simulink model "Simulink_Encoder"  (R2023b)
settings: Solver=FixedStepAuto  StartTime=0.0  StopTime=10  RelTol=1e-3
undefined symbols (not defined in the file): DiscIntNeverNeededParam
libraries: simulink x3
settings Model: Creator=rodri  LastModifiedBy=rodri

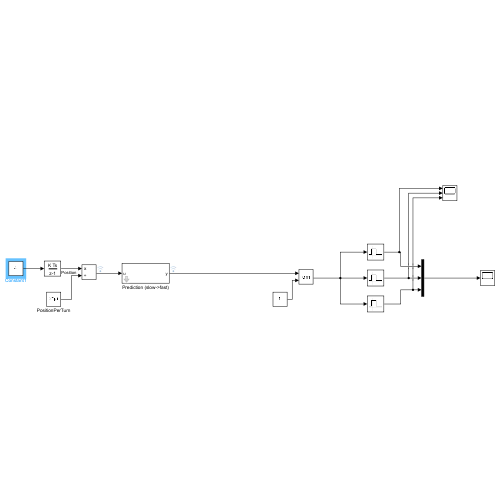
[thumbnail: Simulink's stored preview of the top-level diagram]
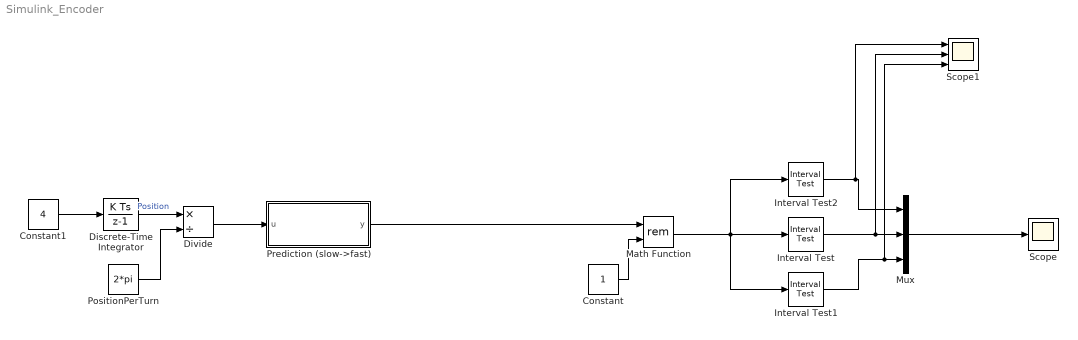
== system Simulink_Encoder ==
  Constant : Constant
  Constant1 : Constant  Value=4  SampleTime=0.1
  Discrete-Time Integrator : DiscreteIntegrator  SampleTime=-1  ICPrevOutput=DiscIntNeverNeededParam  ICPrevScaledInput=DiscIntNeverNeededParam
  Divide : Product  Inputs=*/  RndMeth=Simplest
  Interval Test : simulink/Logic and Bit Operations/Interval Test  IntervalClosedRight=on  uplimit=1  IntervalClosedLeft=on  lowlimit=0.5  OutDataTypeStr=boolean
  Interval Test1 : simulink/Logic and Bit Operations/Interval Test  IntervalClosedRight=on  uplimit=0.125  IntervalClosedLeft=on  lowlimit=0  OutDataTypeStr=boolean
  Interval Test2 : simulink/Logic and Bit Operations/Interval Test  IntervalClosedRight=on  uplimit=0.5  IntervalClosedLeft=on  lowlimit=0  OutDataTypeStr=boolean
  Math Function : Math  Operator=rem
  Mux : Mux  Inputs=3
  PositionPerTurn : Constant  Value=2*pi
  Prediction (slow->fast) : Subsystem  mask(Prediction (slow->fast)){h2=0.1, h1=0.001}
      mask prompts: h2 "physmod:simscape:couplers:SimscapeNetworkCouplersLib:PortUDiscreteSampleTimes_MP"; h1 "physmod:simscape:couplers:SimscapeNetworkCouplersLib:PortYDiscreteSampleTimes_MP"
      mask help: physmod:simscape:couplers:SimscapeNetworkCouplersLib:Predictionslowfast_MD
      mask Help: web([docroot '/simscape/ref/predictionslowfast.html'])
      mask DialogControl h2 Prompt: Port u discrete sample time (s)
      mask DialogControl h1 Prompt: Port y discrete sample time (s)
  Scope : Scope
  Scope1 : Scope  NumInputPorts=3
  wires:
  Mux/1 -> Scope/1
  PositionPerTurn/1 -> Divide/2
  Discrete-Time Integrator/1 -> Divide/1  "Position"
  Constant/1 -> Math Function/2
  Prediction (slow->fast)/1(y) -> Math Function/1
  Math Function/1 -> Interval Test1/1, Interval Test/1, Interval Test2/1
  Interval Test2/1 -> Scope1/1, Mux/1
  Interval Test/1 -> Scope1/2, Mux/2
  Interval Test1/1 -> Scope1/3, Mux/3
  Divide/1 -> Prediction (slow->fast)/1(u)
  Constant1/1 -> Discrete-Time Integrator/1

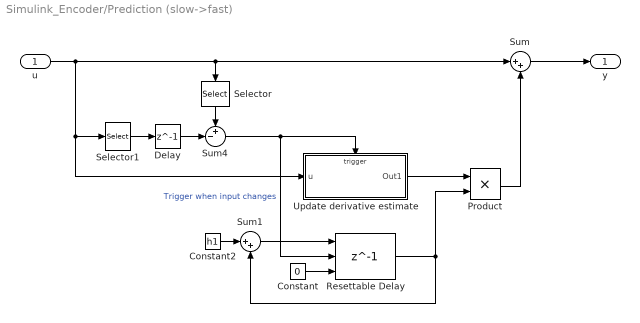
== system Simulink_Encoder/Prediction (slow->fast) ==
  u : Inport
  Constant : Constant  Value=0  SampleTime=h1
  Constant2 : Constant  Value=h1  SampleTime=h1
  "Delay " : Delay  DelayLength=1  SampleTime=h1
  Product : Product
  Resettable Delay : Delay  DelayLength=1  InitialConditionSource=Input port  ExternalReset=Rising  SampleTime=h1
      settings: InputPortMap=u0,r5,p4
  Selector : Selector  IndexOptions=Index vector (dialog)  Indices=1  OutputSizes=1
  Selector1 : Selector  IndexOptions=Index vector (dialog)  Indices=1  OutputSizes=1
  Sum : Sum  Inputs=|++
  Sum1 : Sum  Inputs=|++
  Sum4 : Sum  Inputs=+-|
  Update derivative estimate : Subsystem  TreatAsAtomicUnit=on
  y : Outport
  wires:
  Selector1/1 -> "Delay "/1
  Selector/1 -> Sum4/1
  Product/1 -> Sum/2
  Sum/1 -> y/1
  Constant/1 -> Resettable Delay/3
  Constant2/1 -> Sum1/1
  Resettable Delay/1 -> Sum1/2, Product/2
  Sum1/1 -> Resettable Delay/1
  Sum4/1 -> Resettable Delay/2, Update derivative estimate/Trigger  "Trigger when input changes"
  "Delay "/1 -> Sum4/2
  u/1 -> Sum/1, Selector/1, Update derivative estimate/1(u), Selector1/1
  Update derivative estimate/1(Out1) -> Product/1

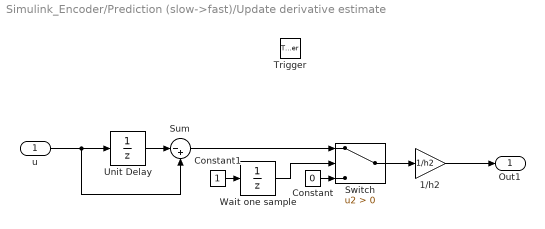
== system Simulink_Encoder/Prediction (slow->fast)/Update derivative estimate ==
  u : Inport
  Trigger : TriggerPort  VariantControl=(inherit)
  1/h2 : Gain  Gain=1/h2
  Constant : Constant  Value=0  SampleTime=-1
  Constant1 : Constant  SampleTime=-1
  Sum : Sum  Inputs=|-+
  Switch : Switch  Criteria=u2 > Threshold  SaturateOnIntegerOverflow=off  InputSameDT=off
  Unit Delay : UnitDelay  SampleTime=-1  HasFrameUpgradeWarning=on
  Wait one sample : UnitDelay  SampleTime=-1  HasFrameUpgradeWarning=on
  Out1 : Outport
  wires:
  Unit Delay/1 -> Sum/1
  u/1 -> Unit Delay/1, Sum/2
  1/h2/1 -> Out1/1
  Switch/1 -> 1/h2/1
  Sum/1 -> Switch/1
  Constant/1 -> Switch/3
  Wait one sample/1 -> Switch/2
  Constant1/1 -> Wait one sample/1
